simulink model "AltrFir32"  (Simulink 6.3)
settings: Solver=FixedStepDiscrete  SolverMode=SingleTasking  StartTime=0.0  StopTime=3000  RelTol=1e-3
PreLoadFcn:
  | close all
  | clear all
  | FilterOrder = 32
  | InputBitWidth = 8
  | LowPassFreqBand = [0 0.1 0.2 1];
  | LowPassMagnBand = [1 0.9 0.0001 0.0001];
  | 
  | FlCoef = firls(FilterOrder,LowPassFreqBand,LowPassMagnBand);
  | 
  | CoefBitWidth = InputBitWidth + ceil(log2((max(abs(FlCoef))/min(abs(FlCoef)))))
  | 
  | ScalingFactor = (2^(CoefBitWidth-1))-1;
  | FpCoef = fix(ScalingFactor * FlCoef);
  | plot(FpCoef,'o');
  | title('Fixed-point scaled coefficient value');
  | ImpulseData = zeros(1,1000);
  | ImpulseData(1) = 100;
  | h = conv(ImpulseData,FpCoef);
  | fftplot(h);
  | title('FIR Frequency response');
  | FirSamplingPeriod=1;
InitFcn:
  | %% DSPBuilder Start
  | alt_dspbuilder_update_model(bdroot)
  | %% DSPBuilder End
libraries: allblocks_alteradspbuilder2 x41, simulink_extras x1
settings Model: Creator=mjervis  LastModifiedBy=LKONG
settings DataIOCC: SignalLoggingName=sigsOut
settings OptimizationCC: BooleanDataType=off  InlineInvariantSignals=on
settings DebuggingCC: SolverPrmCheckMsg=none
settings HardwareCC: TargetUnknown=on

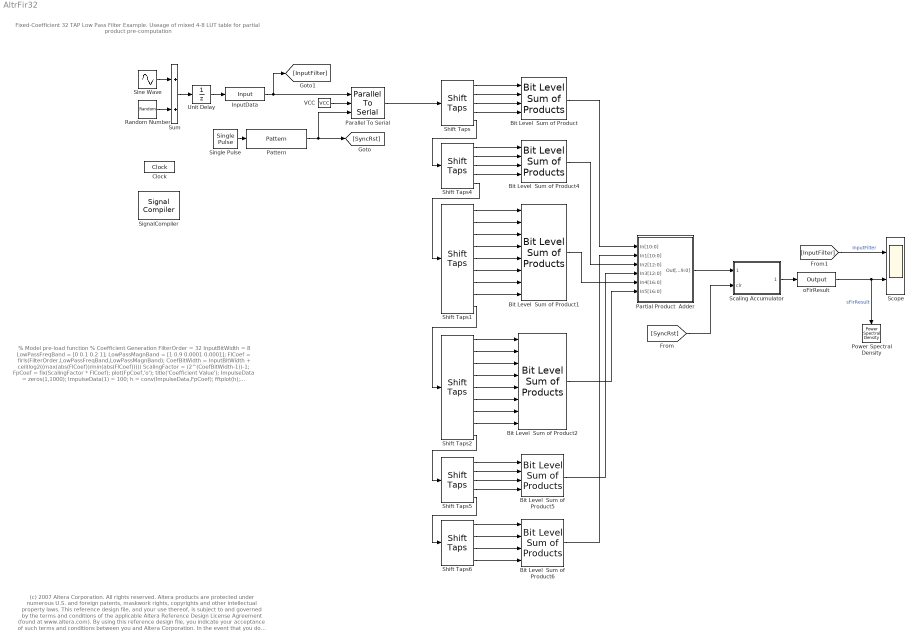
== system AltrFir32 ==
  note: Fixed-Coefficient 32 TAP Low Pass Filter Example.
      | Useage of mixed 4-8 LUT table for partial product pre-computation
  note: % Model pre-load function
      | % Coefficient Generation
      | FilterOrder = 32
      | InputBitWidth = 8
      | LowPassFreqBand = [0 0.1 0.2 1];
      | LowPassMagnBand = [1 0.9 0.0001 0.0001];
      |
      | FlCoef = firls(FilterOrder,LowPassFreqBand,LowPassMagnBand);
      |
      | CoefBitWidth = InputBitWidth + ceil(log2((max(abs(FlCoef))/min(abs(FlCoef)))))
      | ScalingFactor = (2^(CoefBitWidth-1))-1;
      |
      | FpCoef = fix(ScalingFactor * FlCoef);
      |
      | plot(FpCoef,'o');
      | title('Coefficient Value');
      | ImpulseData = zeros(1,1000);
      | ImpulseData(1) = 100;
      | h = conv(ImpulseData,FpCoef);
      | fftplot(h);
      | title('Frequency response');
      | FirSamplingPeriod=1;
  note: (c) 2007 Altera Corporation. All rights reserved.  Altera products are protected under numerous U.S. and foreign patents, maskwork rights, copyrights and other intellectual property laws.
      | This reference design file, and your use thereof, is subject to and governed by the terms and conditions of the applicable Altera Reference Design License Agreement (found at www.altera.com).
      | By using this reference design file, you indicate your acceptance of such terms and conditions between you and Altera Corporation.
      | In the event that you do not agree with such terms and conditions, you may not use the reference design file and please promptly destroy any copies you have made.
      | This reference design file being provided on an "as-is" basis and as an accommodation and therefore all warranties, representations or guarantees of any kind (whether express, implied or statutory)
      | including, without limitation, warranties of merchantability, non-infringement, or fitness for a particular purpose, are specifically disclaimed.
      | By making this reference design file available, Altera expressly does not recommend, suggest or require that this reference design file be used in combination with any other product not provided by Altera
  Bit Level  Sum of Product : allblocks_alteradspbuilder2/Bit Level Sum of Products  number_of_coefficients=4  BusType=Signed Integer  bwl=9  bwr=0  coefficients=[FpCoef(1:4)]  register_inputs=off  use_ena=off  use_sclr=off
  Bit Level  Sum of Product1 : allblocks_alteradspbuilder2/Bit Level Sum of Products  number_of_coefficients=8  BusType=Signed Integer  bwl=14  bwr=0  coefficients=[FpCoef(9:16)]  register_inputs=off  use_ena=off  use_sclr=off
  Bit Level  Sum of Product2 : allblocks_alteradspbuilder2/Bit Level Sum of Products  number_of_coefficients=8  BusType=Signed Integer  bwl=14  bwr=0  coefficients=[FpCoef(17:24)]  register_inputs=off  use_ena=off  use_sclr=off
  Bit Level  Sum of Product4 : allblocks_alteradspbuilder2/Bit Level Sum of Products  number_of_coefficients=4  BusType=Signed Integer  bwl=11  bwr=0  coefficients=[FpCoef(5:8)]  register_inputs=off  use_ena=off  use_sclr=off
  Bit Level  Sum of Product5 : allblocks_alteradspbuilder2/Bit Level Sum of Products  number_of_coefficients=4  BusType=Signed Integer  bwl=11  bwr=0  coefficients=[FpCoef(25:28)]  register_inputs=off  use_ena=off  use_sclr=off
  Bit Level  Sum of Product6 : allblocks_alteradspbuilder2/Bit Level Sum of Products  number_of_coefficients=4  BusType=Signed Integer  bwl=9  bwr=0  coefficients=[FpCoef(29:32)]  register_inputs=off  use_ena=off  use_sclr=off
  Clock : allblocks_alteradspbuilder2/Clock  ClockPeriod=20  ClockPeriodUnit=ns  SampleTime=1  SimulationStartCycle=5  PhaseOffset=0  Reset=aclr  ResetType=Active Low  Export=off
  InputData : allblocks_alteradspbuilder2/Input  iofile=d:\wsTrunk\workspace\Documentation\DesignExamples\Demos\Filters\DA32\tb_AltrFir32\AltrFir32_InputData.salt  BusType=Signed Integer  bwl=8  bwr=0  SpecifyClock=off  PORTTYPE=Input
  Parallel To Serial : allblocks_alteradspbuilder2/Parallel To Serial  BusType=Signed Integer  bwl=8  bwr=0  msbfirsttext=LSB First  msbfirst=0  repeatlastbit=on  use_ena=on  use_sclr=off
  Partial Product  Adder : Subsystem
      mask Type: SubSystem AlteraBlockSet
  Pattern : allblocks_alteradspbuilder2/Pattern  Sequence=10000000  SpecifyClock=off  use_ena=on  use_sclr=off
  Power Spectral Density : simulink_extras/Additional Sinks/Power Spectral Density  Orientation=down  npts=256  fftpts=1024  HowOften=64  sampleT=8
  Random Number : RandomNumber  Variance=50  SampleTime=1
  Scaling Accumulator : Subsystem
      mask Type: SubSystem AlteraBlockSet
  Scope : Scope  NumInputPorts=2
      settings: TimeRange=3000  YMin=-150~-30  YMax=150~30
  Shift Taps : allblocks_alteradspbuilder2/Shift Taps  number_of_taps=4  tap_distance=8  use_shiftout=on  use_ena=off  use_sclr=off  use_dedicated_circuitry=on  ram_type=AUTO
  Shift Taps1 : allblocks_alteradspbuilder2/Shift Taps  number_of_taps=8  tap_distance=8  use_shiftout=on  use_ena=off  use_sclr=off  use_dedicated_circuitry=on  ram_type=AUTO
  Shift Taps2 : allblocks_alteradspbuilder2/Shift Taps  number_of_taps=8  tap_distance=8  use_shiftout=on  use_ena=off  use_sclr=off  use_dedicated_circuitry=on  ram_type=AUTO
  Shift Taps4 : allblocks_alteradspbuilder2/Shift Taps  number_of_taps=4  tap_distance=8  use_shiftout=on  use_ena=off  use_sclr=off  use_dedicated_circuitry=on  ram_type=AUTO
  Shift Taps5 : allblocks_alteradspbuilder2/Shift Taps  number_of_taps=4  tap_distance=8  use_shiftout=on  use_ena=off  use_sclr=off  use_dedicated_circuitry=on  ram_type=AUTO
  Shift Taps6 : allblocks_alteradspbuilder2/Shift Taps  number_of_taps=4  tap_distance=8  use_shiftout=off  use_ena=off  use_sclr=off  use_dedicated_circuitry=on  ram_type=AUTO
  SignalCompiler : allblocks_alteradspbuilder2/Signal Compiler  DeviceFamily=Stratix IV  DeviceName=AUTO  EnableSignalTap=off  SignalTapDepth=128  UseBoardBlock=off  StpUseDefaultClock=on  StpClock=clock
  Sine Wave : Sin  SineType=Sample based  Amplitude=100  Samples=100  SampleTime=8
  "Single Pulse " : allblocks_alteradspbuilder2/Single Pulse  signal_type=Step Up  impulse_width=1  delay=1  SpecifyClock=off  use_ena=off  use_sclr=off
  Sum : Sum  SaturateOnIntegerOverflow=on  InputSameDT=on
  Unit Delay : UnitDelay
  VCC : allblocks_alteradspbuilder2/VCC  SpecifyClock=off
  oFirResult : allblocks_alteradspbuilder2/Output  iofile=d:\wsTrunk\workspace\Documentation\DesignExamples\Demos\Filters\DA32\tb_AltrFir32\AltrFir32_oFirResult.capture  BusType=Signed Integer  bwl=11  bwr=0  PORTTYPE=Output
  wires:
  Shift Taps1/1 -> Bit Level  Sum of Product1/1
  Shift Taps1/2 -> Bit Level  Sum of Product1/2
  Shift Taps1/3 -> Bit Level  Sum of Product1/3
  Shift Taps1/4 -> Bit Level  Sum of Product1/4
  Shift Taps1/5 -> Bit Level  Sum of Product1/5
  Shift Taps1/6 -> Bit Level  Sum of Product1/6
  Shift Taps1/7 -> Bit Level  Sum of Product1/7
  Shift Taps1/8 -> Bit Level  Sum of Product1/8
  Shift Taps2/1 -> Bit Level  Sum of Product2/1
  Shift Taps2/2 -> Bit Level  Sum of Product2/2
  Shift Taps2/3 -> Bit Level  Sum of Product2/3
  Shift Taps2/4 -> Bit Level  Sum of Product2/4
  Shift Taps2/5 -> Bit Level  Sum of Product2/5
  Shift Taps2/6 -> Bit Level  Sum of Product2/6
  Shift Taps2/7 -> Bit Level  Sum of Product2/7
  Shift Taps2/8 -> Bit Level  Sum of Product2/8
  Shift Taps1/9 -> Shift Taps2/1
  Parallel To Serial/1 -> Shift Taps/1
  "Single Pulse "/1 -> Pattern/1
  Pattern/1 -> [SyncRst], Parallel To Serial/3
  [SyncRst] -> Scaling Accumulator/2(clr)
  Partial Product  Adder/1(Out[19:0]) -> Scaling Accumulator/1(In[19:0])
  Shift Taps/1 -> Bit Level  Sum of Product/1
  Shift Taps/2 -> Bit Level  Sum of Product/2
  Shift Taps/3 -> Bit Level  Sum of Product/3
  Shift Taps/4 -> Bit Level  Sum of Product/4
  Shift Taps4/1 -> Bit Level  Sum of Product4/1
  Shift Taps4/2 -> Bit Level  Sum of Product4/2
  Shift Taps4/3 -> Bit Level  Sum of Product4/3
  Shift Taps4/4 -> Bit Level  Sum of Product4/4
  Shift Taps/5 -> Shift Taps4/1
  Shift Taps4/5 -> Shift Taps1/1
  Shift Taps5/1 -> Bit Level  Sum of Product5/1
  Shift Taps5/2 -> Bit Level  Sum of Product5/2
  Shift Taps5/3 -> Bit Level  Sum of Product5/3
  Shift Taps5/4 -> Bit Level  Sum of Product5/4
  Shift Taps6/1 -> Bit Level  Sum of Product6/1
  Shift Taps6/2 -> Bit Level  Sum of Product6/2
  Shift Taps6/3 -> Bit Level  Sum of Product6/3
  Shift Taps6/4 -> Bit Level  Sum of Product6/4
  Shift Taps5/5 -> Shift Taps6/1
  Shift Taps2/9 -> Shift Taps5/1
  Bit Level  Sum of Product5/1 -> Partial Product  Adder/4(In3[12:0])
  Bit Level  Sum of Product/1 -> Partial Product  Adder/1(In[10:0])
  Bit Level  Sum of Product6/1 -> Partial Product  Adder/2(In1[10:0])
  Bit Level  Sum of Product4/1 -> Partial Product  Adder/3(In2[12:0])
  Bit Level  Sum of Product1/1 -> Partial Product  Adder/5(In4[16:0])
  Bit Level  Sum of Product2/1 -> Partial Product  Adder/6(In5[16:0])
  VCC/1 -> Parallel To Serial/2
  InputData/1 -> Parallel To Serial/1, [InputFilter]
  Unit Delay/1 -> InputData/1
  [InputFilter] -> Scope/1  "InputFilter"
  oFirResult/1 -> Scope/2, Power Spectral Density/1  "sFirResult"
  Sum/1 -> Unit Delay/1
  Sine Wave/1 -> Sum/1
  Random Number/1 -> Sum/2
  Scaling Accumulator/1(Out[10:0]) -> oFirResult/1

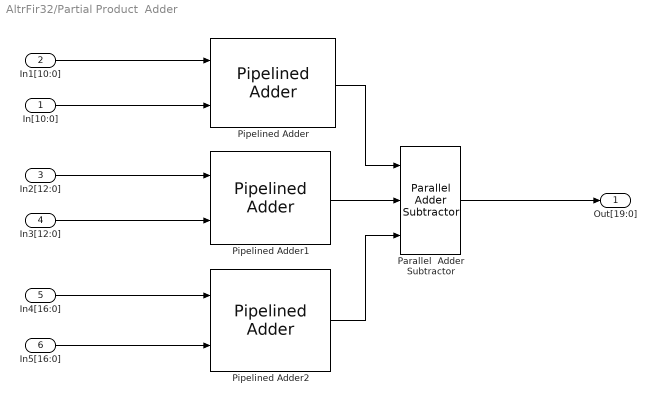
== system AltrFir32/Partial Product  Adder ==
  In[10:0] : Inport
  In1[10:0] : Inport  Port=2
  In2[12:0] : Inport  Port=3
  In3[12:0] : Inport  Port=4
  In4[16:0] : Inport  Port=5
  In5[16:0] : Inport  Port=6
  Parallel  Adder Subtractor : allblocks_alteradspbuilder2/Parallel Adder Subtractor  number_of_inputs=3  direction=++  use_pipeline=on  phase_selection=1  use_ena=off  use_aclr=off
  Pipelined Adder : allblocks_alteradspbuilder2/Pipelined Adder  BusType=Signed Integer  bwl=12  bwr=0  pipeline=2  AddSubDirection=ADD  use_cin=off  use_ovl=off  use_addsub=off  use_ena=off  use_aclr=off
  Pipelined Adder1 : allblocks_alteradspbuilder2/Pipelined Adder  BusType=Signed Integer  bwl=14  bwr=0  pipeline=2  AddSubDirection=ADD  use_cin=off  use_ovl=off  use_addsub=off  use_ena=off  use_aclr=off
  Pipelined Adder2 : allblocks_alteradspbuilder2/Pipelined Adder  BusType=Signed Integer  bwl=18  bwr=0  pipeline=2  AddSubDirection=ADD  use_cin=off  use_ovl=off  use_addsub=off  use_ena=off  use_aclr=off
  Out[19:0] : Outport
  wires:
  In[10:0]/1 -> Pipelined Adder/2
  In1[10:0]/1 -> Pipelined Adder/1
  In2[12:0]/1 -> Pipelined Adder1/1
  In3[12:0]/1 -> Pipelined Adder1/2
  In4[16:0]/1 -> Pipelined Adder2/1
  In5[16:0]/1 -> Pipelined Adder2/2
  Pipelined Adder/1 -> Parallel  Adder Subtractor/1
  Pipelined Adder1/1 -> Parallel  Adder Subtractor/2
  Pipelined Adder2/1 -> Parallel  Adder Subtractor/3
  Parallel  Adder Subtractor/1 -> Out[19:0]/1

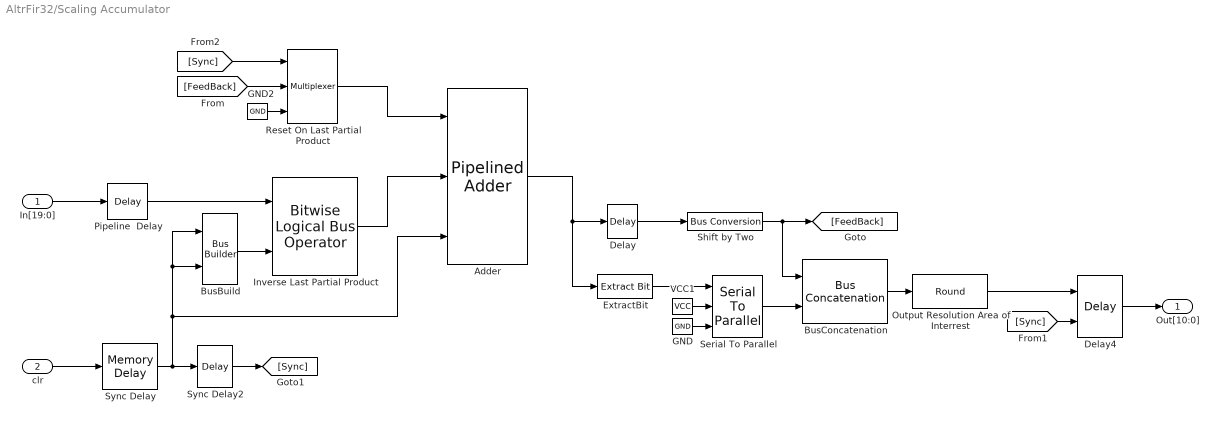
== system AltrFir32/Scaling Accumulator ==
  In[19:0] : Inport
  clr : Inport  Port=2
  Adder : allblocks_alteradspbuilder2/Pipelined Adder  BusType=Signed Integer  bwl=21  bwr=0  pipeline=0  AddSubDirection=ADD  use_cin=on  use_ovl=off  use_addsub=off  use_ena=on  use_aclr=on
  BusBuild : allblocks_alteradspbuilder2/Bus Builder  BusType=Signed Integer  bwl=2  bwr=0
  BusConcatenation : allblocks_alteradspbuilder2/Bus Concatenation  isSigned=on  awidth=20  bwidth=8
  Delay : allblocks_alteradspbuilder2/Delay  pipeline=1  ClockPhase=1  use_ena=off  use_sclr=off  use_init=off  reset_value=1
  Delay4 : allblocks_alteradspbuilder2/Delay  pipeline=1  ClockPhase=1  use_ena=on  use_sclr=off  use_init=off  reset_value=1
  ExtractBit : allblocks_alteradspbuilder2/Extract Bit  BusType=Signed Fractional  bwl=21  bwr=0  bitToSelect=0
  GND : allblocks_alteradspbuilder2/GND  SpecifyClock=off
  GND2 : allblocks_alteradspbuilder2/GND  SpecifyClock=off
  Inverse Last Partial Product : allblocks_alteradspbuilder2/Bitwise Logical Bus Operator  BusType=Signed Integer  bwl=20  bwr=0  LogicalOperator=XOR
  Output Resolution Area of Interrest : allblocks_alteradspbuilder2/Round  BusType=Signed Integer  bwl=28  bwr=0  bitsToRemove=17  roundMode=TRUNCATE_LOW  userRoundMode=Truncate  pipeline=off
  Pipeline  Delay : allblocks_alteradspbuilder2/Delay  pipeline=1  ClockPhase=1  use_ena=off  use_sclr=off  use_init=off  reset_value=1
  Reset On Last Partial Product : allblocks_alteradspbuilder2/Multiplexer  numInputs=2  pipeline=0  oneHot=off  use_ena=off  use_aclr=off
  Serial To Parallel : allblocks_alteradspbuilder2/Serial To Parallel  BusType=Unsigned Integer  bwl=8  bwr=0  msbfirsttext=LSB First  msbfirst=0  use_ena=on  use_sclr=on
  Shift by Two : allblocks_alteradspbuilder2/Bus Conversion  BusType=Signed Integer  ibwl=21  ibwr=0  bwl=20  bwr=0  bitToConnectToOutputLSB=1  round=off  saturate=off
  Sync Delay : allblocks_alteradspbuilder2/Memory Delay  BusType=Inferred  bwl=8  bwr=0  pipeline=13  ram_type=AUTO  use_ena=off  use_sclr=off
  Sync Delay2 : allblocks_alteradspbuilder2/Delay  pipeline=1  ClockPhase=1  use_ena=off  use_sclr=off  use_init=off  reset_value=1
  VCC1 : allblocks_alteradspbuilder2/VCC  SpecifyClock=off
  Out[10:0] : Outport
  wires:
  clr/1 -> Sync Delay/1
  In[19:0]/1 -> Pipeline  Delay/1
  Delay/1 -> Shift by Two/1
  Shift by Two/1 -> BusConcatenation/1, [FeedBack]
  VCC1/1 -> Serial To Parallel/2
  Serial To Parallel/1 -> BusConcatenation/2
  GND/1 -> Serial To Parallel/3
  Delay4/1 -> Out[10:0]/1
  BusConcatenation/1 -> Output Resolution Area of Interrest/1
  ExtractBit/1 -> Serial To Parallel/1
  Reset On Last Partial Product/1 -> Adder/1
  GND2/1 -> Reset On Last Partial Product/3
  [FeedBack] -> Reset On Last Partial Product/2
  [Sync] -> Delay4/2
  [Sync] -> Reset On Last Partial Product/1
  Adder/1 -> Delay/1, ExtractBit/1
  Sync Delay/1 -> Sync Delay2/1, BusBuild/2, BusBuild/1, Adder/3
  Inverse Last Partial Product/1 -> Adder/2
  Pipeline  Delay/1 -> Inverse Last Partial Product/1
  Sync Delay2/1 -> [Sync]
  Output Resolution Area of Interrest/1 -> Delay4/1
  BusBuild/1 -> Inverse Last Partial Product/2
